simulink subsystem "driver"  (R2024b)
settings: Solver=VariableStepAuto  StartTime=0.0  StopTime=10.0  RelTol=1e-3
values from neighbouring files (symbols this model uses):
  Ts = 1e-2    (= 0.01)    [balrob_params.m]
undefined symbols (not defined in the file or in its folder): drv
settings Model: Creator=Sofia  LastModifiedBy=Davide Pillon

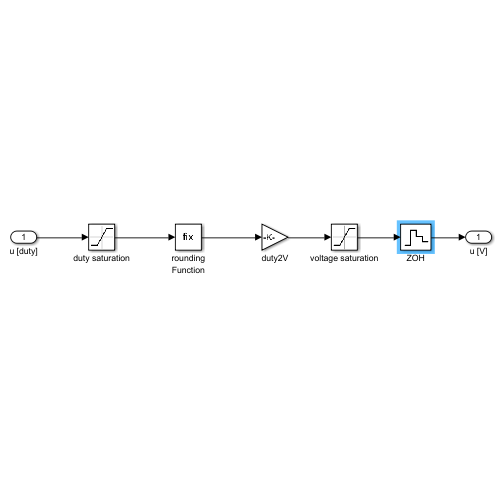
[thumbnail: Simulink's stored preview of the top-level diagram]
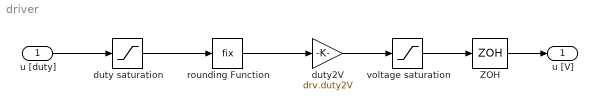
== system driver ==
  u [duty] : Inport
  ZOH : ZeroOrderHold  SampleTime=Ts
  duty saturation : Saturate  UpperLimit=drv.dutymax  LowerLimit=-drv.dutymax
  duty2V : Gain  Gain=drv.duty2V
  rounding Function : Rounding  Operator=fix
  voltage saturation : Saturate  UpperLimit=drv.Vbus  LowerLimit=-drv.Vbus
  u [V] : Outport
  wires:
  rounding Function/1 -> duty2V/1
  ZOH/1 -> u [V]/1
  u [duty]/1 -> duty saturation/1
  voltage saturation/1 -> ZOH/1
  duty2V/1 -> voltage saturation/1
  duty saturation/1 -> rounding Function/1
